simulink model "two_time_domains"  (R2025b)
settings: Solver=ode23tb  StartTime=0.0  StopTime=simlength  MaxStep=tc
undefined symbols (not defined in the file): D1, omega_base, P, time_gain_afe_module_1, time_gain_afe_module_2, time_gain_inv_module_2, trgo_th_generator, ts_afe, ts_inv
settings Model: Creator=dbagn  LastModifiedBy=dbagn
settings SolverCC: NumberNewtonIterations=3.0  ZeroCrossControl=DisableAll  AlgebraicLoopSolver=TrustRegion  SolverResetMethod=Robust  AutoInsertRateTranBlk=on
settings DataIOCC: SaveOutput=off  SignalLogging=off  DSMLogging=off  SaveTime=off  ReturnWorkspaceOutputs=off
settings OptimizationCC: ReuseModelBlockBuffer=off
settings DebuggingCC: UnconnectedInputMsg=warning  UnconnectedOutputMsg=warning  UnconnectedLineMsg=warning
settings ModelReferenceCC: UpdateModelReferenceTargets=Force  EnableRefExpFcnMdlSchedulingChecks=on  ParallelModelReferenceMATLABWorkerInit=Copy Base Workspace
settings SFSimCC: CustomCodeUndefinedFunction=ThrowError  DefaultCustomCodeDeterministicFunctions=All
settings RTWCC: GPUComputeCapability=3.5  DLArmComputeVersion=19.05

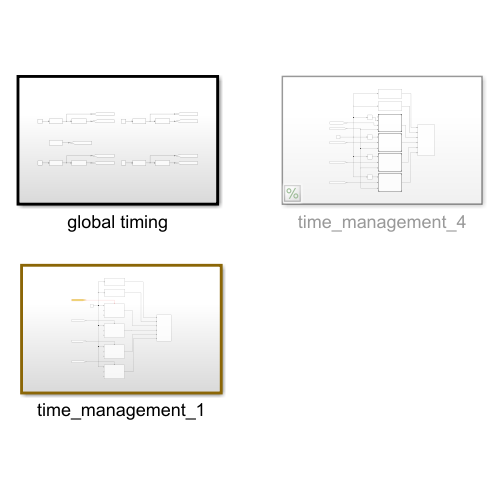
[thumbnail: Simulink's stored preview of the top-level diagram]
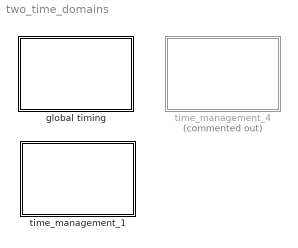
== system two_time_domains ==
  global timing : Subsystem
  time_management_1 : Subsystem
  time_management_4 : Subsystem  Commented=on

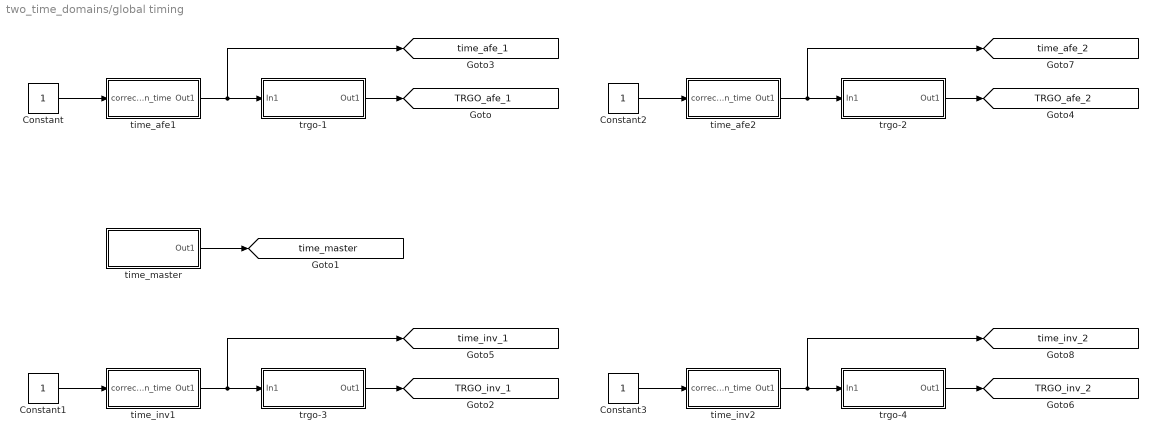
== system two_time_domains/global timing ==
  Constant{,1..3} (4 alike) : Constant
  time_afe1 : Subsystem  mask{k=time_gain_afe_module_1}
      mask prompts: k "Time Gain"
      mask Display:
      | disp('time-gen');
      | port_label('input', 1, 'crt');
      | port_label('output', 1, 'tout');
  time_afe2 : Subsystem  mask{k=time_gain_afe_module_2}
      mask prompts: k "Time Gain"
      mask Display:
      | disp('time-gen');
      | port_label('input', 1, 'crt');
      | port_label('output', 1, 'tout');
  time_inv1 : Subsystem  mask{k=time_gain_afe_module_1}
      mask prompts: k "Time Gain"
      mask Display:
      | disp('time-gen');
      | port_label('input', 1, 'crt');
      | port_label('output', 1, 'tout');
  time_inv2 : Subsystem  mask{k=time_gain_inv_module_2}
      mask prompts: k "Time Gain"
      mask Display:
      | disp('time-gen');
      | port_label('input', 1, 'crt');
      | port_label('output', 1, 'tout');
  time_master : Subsystem  mask{k=1}
      mask prompts: k "Time Gain"
      mask Display:
      | disp('master');
      | port_label('output', 1, 'time');
  trgo-1 : Subsystem  mask{samplig_time=ts_afe}
      mask prompts: samplig_time "Sampling Time"
      mask Display: disp('TRGO Generator');
  trgo-2 : Subsystem  mask{samplig_time=ts_afe}
      mask prompts: samplig_time "Sampling Time"
      mask Display: disp('TRGO Generator');
  trgo-3 : Subsystem  mask{samplig_time=ts_inv}
      mask prompts: samplig_time "Sampling Time"
      mask Display: disp('TRGO Generator');
  trgo-4 : Subsystem  mask{samplig_time=ts_inv}
      mask prompts: samplig_time "Sampling Time"
      mask Display: disp('TRGO Generator');
  tag scope: TRGO_afe_1=global, TRGO_afe_2=global, TRGO_inv_1=global, TRGO_inv_2=global, time_afe_1=global, time_afe_2=global, time_inv_1=global, time_inv_2=global, time_master=global
  wires:
  Constant/1 -> time_afe1/1(correction_time)
  time_afe1/1(Out1) -> [time_afe_1], trgo-1/1(In1)
  trgo-1/1(Out1) -> [TRGO_afe_1]
  trgo-2/1(Out1) -> [TRGO_afe_2]
  time_afe2/1(Out1) -> trgo-2/1(In1), [time_afe_2]
  Constant2/1 -> time_afe2/1(correction_time)
  time_master/1(Out1) -> [time_master]
  Constant3/1 -> time_inv2/1(correction_time)
  time_inv2/1(Out1) -> [time_inv_2], trgo-4/1(In1)
  trgo-4/1(Out1) -> [TRGO_inv_2]
  trgo-3/1(Out1) -> [TRGO_inv_1]
  time_inv1/1(Out1) -> trgo-3/1(In1), [time_inv_1]
  Constant1/1 -> time_inv1/1(correction_time)

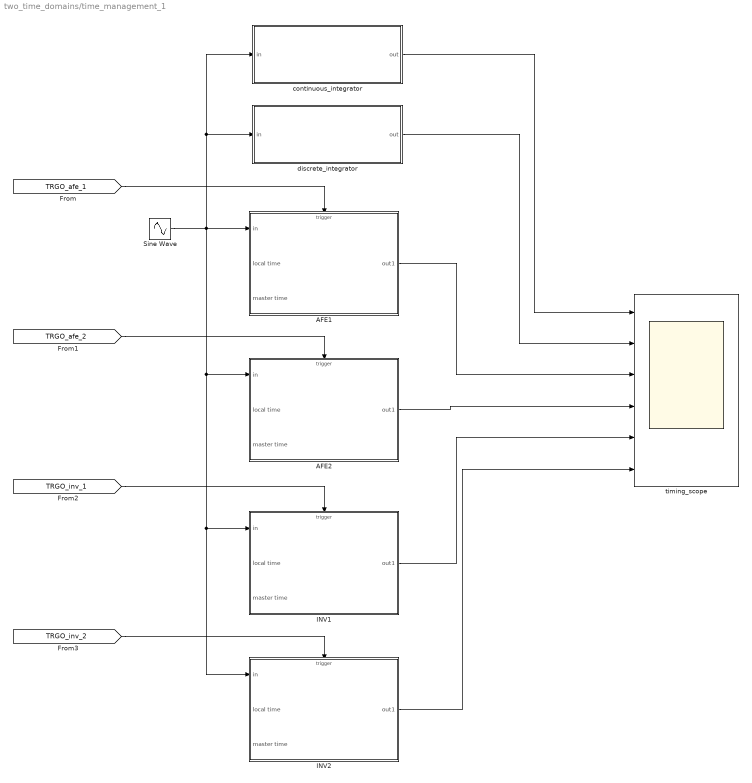
== system two_time_domains/time_management_1 ==
  AFE1 : Subsystem
  AFE2 : Subsystem
  INV1 : Subsystem
  INV2 : Subsystem
  Sine Wave : Sin  Frequency=omega_base  SampleTime=0
  continuous_integrator : Subsystem
  discrete_integrator : Subsystem
  timing_scope : Scope  NumInputPorts=6
      settings: SampleTime=tc  ActiveDisplayYMinimum=-0.51142077441090428  ActiveDisplayYMaximum=2.52734484585139
  wires:
  [TRGO_afe_1] -> AFE1/Trigger
  [TRGO_afe_2] -> AFE2/Trigger
  Sine Wave/1 -> discrete_integrator/1(in), continuous_integrator/1(in), AFE1/1(in), AFE2/1(in), INV2/1(in), INV1/1(in)
  [TRGO_inv_2] -> INV2/Trigger
  [TRGO_inv_1] -> INV1/Trigger
  AFE1/1(out1) -> timing_scope/3
  AFE2/1(out1) -> timing_scope/4
  INV1/1(out1) -> timing_scope/5
  INV2/1(out1) -> timing_scope/6
  discrete_integrator/1(out) -> timing_scope/2
  continuous_integrator/1(out) -> timing_scope/1

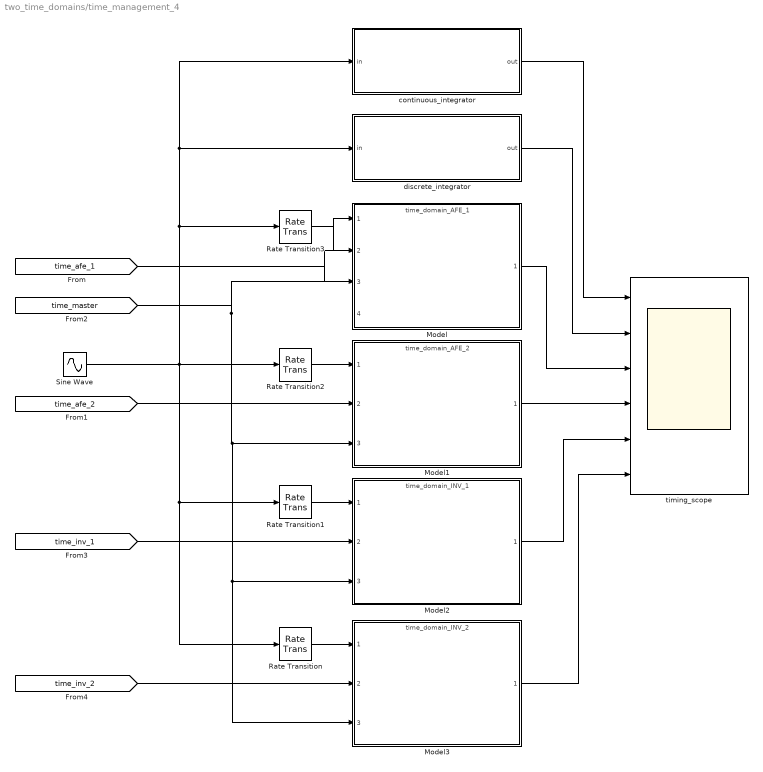
== system two_time_domains/time_management_4 ==
  Model : ModelReference  ModelNameDialog=time_domain_AFE_1  SimulationMode=Normal  ScheduleRates=on  CachedPortDiscreteRates=[0.00014000000000000001]  ModelEventPortInfo=P:D1[0.00014000000000000001][0][0]  ModelReferenceVersion=1.18  CommunicationStepSize=ts_afe_1
  Model1 : ModelReference  ModelNameDialog=time_domain_AFE_2  SimulationMode=Normal  ModelReferenceVersion=1.16  CommunicationStepSize=ts_afe_2
  Model2 : ModelReference  ModelNameDialog=time_domain_INV_1  SimulationMode=Normal  ModelReferenceVersion=1.19  CommunicationStepSize=ts_afe_1
  Model3 : ModelReference  ModelNameDialog=time_domain_INV_2  SimulationMode=Normal  ModelReferenceVersion=1.18  CommunicationStepSize=ts_afe_2
  Rate Transition : RateTransition  OutPortSampleTime=ts_inv_2
  Rate Transition1 : RateTransition  OutPortSampleTime=ts_inv_1
  Rate Transition2 : RateTransition  OutPortSampleTime=ts_afe_2
  Rate Transition3 : RateTransition  OutPortSampleTime=ts_afe_1
  Sine Wave : Sin  Frequency=omega_base  SampleTime=0
  continuous_integrator : Subsystem
  discrete_integrator : Subsystem
  timing_scope : Scope  NumInputPorts=6
      settings: SampleTime=tc  ActiveDisplayYMinimum=-0.24998930779814185  ActiveDisplayYMaximum=2.2499037701832774
  wires:
  Model/1 -> timing_scope/3
  Model1/1 -> timing_scope/4
  discrete_integrator/1(out) -> timing_scope/2
  [time_afe_1] -> Model/2
  [time_afe_2] -> Model1/2
  [time_master] -> Model3/3, Model2/3, Model1/3, Model/3
  Model2/1 -> timing_scope/5
  Model3/1 -> timing_scope/6
  Sine Wave/1 -> Rate Transition/1, Rate Transition1/1, discrete_integrator/1(in), continuous_integrator/1(in), Rate Transition3/1, Rate Transition2/1
  Rate Transition/1 -> Model3/1
  Rate Transition1/1 -> Model2/1
  Rate Transition2/1 -> Model1/1
  Rate Transition3/1 -> Model/1
  [time_inv_1] -> Model2/2
  [time_inv_2] -> Model3/2
  continuous_integrator/1(out) -> timing_scope/1

== system two_time_domains/global timing/time_afe1 ==
  correction_time : Inport
  Gain : Gain  Gain=k
  Product : Product
  time_1 : Clock
  Out1 : Outport
  wires:
  time_1/1 -> Gain/1
  Gain/1 -> Product/2
  Product/1 -> Out1/1
  correction_time/1 -> Product/1

== system two_time_domains/global timing/time_afe2 ==
  correction_time : Inport
  Gain : Gain  Gain=k
  Product : Product
  time_1 : Clock
  Out1 : Outport
  wires:
  correction_time/1 -> Product/1
  Product/1 -> Out1/1
  Gain/1 -> Product/2
  time_1/1 -> Gain/1

== system two_time_domains/global timing/time_inv1 ==
  correction_time : Inport
  Gain : Gain  Gain=k
  Product : Product
  time_1 : Clock
  Out1 : Outport
  wires:
  correction_time/1 -> Product/1
  Product/1 -> Out1/1
  Gain/1 -> Product/2
  time_1/1 -> Gain/1

== system two_time_domains/global timing/time_inv2 ==
  correction_time : Inport
  Gain : Gain  Gain=k
  Product : Product
  time_1 : Clock
  Out1 : Outport
  wires:
  time_1/1 -> Gain/1
  Gain/1 -> Product/2
  Product/1 -> Out1/1
  correction_time/1 -> Product/1

== system two_time_domains/global timing/time_master ==
  Gain : Gain  Gain=k
  time_1 : Clock
  Out1 : Outport
  wires:
  Gain/1 -> Out1/1
  time_1/1 -> Gain/1

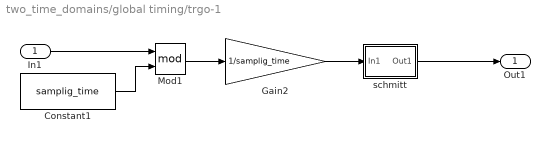
== system two_time_domains/global timing/trgo-1 ==
  In1 : Inport
  Constant1 : Constant  Value=samplig_time
  Gain2 : Gain  Gain=1/samplig_time
  Mod1 : Math  Operator=mod
  schmitt : Subsystem
  Out1 : Outport
  wires:
  Constant1/1 -> Mod1/2
  In1/1 -> Mod1/1
  Mod1/1 -> Gain2/1
  schmitt/1(Out1) -> Out1/1
  Gain2/1 -> schmitt/1(In1)

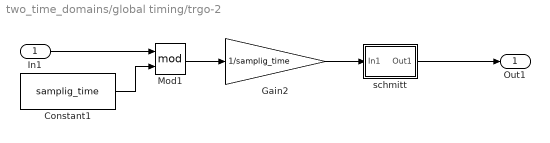
== system two_time_domains/global timing/trgo-2 ==
  In1 : Inport
  Constant1 : Constant  Value=samplig_time
  Gain2 : Gain  Gain=1/samplig_time
  Mod1 : Math  Operator=mod
  schmitt : Subsystem
  Out1 : Outport
  wires:
  Gain2/1 -> schmitt/1(In1)
  schmitt/1(Out1) -> Out1/1
  Mod1/1 -> Gain2/1
  In1/1 -> Mod1/1
  Constant1/1 -> Mod1/2

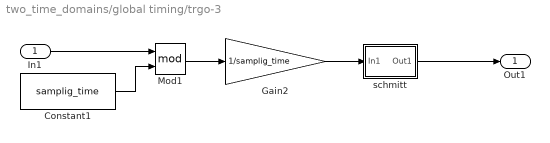
== system two_time_domains/global timing/trgo-3 ==
  In1 : Inport
  Constant1 : Constant  Value=samplig_time
  Gain2 : Gain  Gain=1/samplig_time
  Mod1 : Math  Operator=mod
  schmitt : Subsystem
  Out1 : Outport
  wires:
  Gain2/1 -> schmitt/1(In1)
  schmitt/1(Out1) -> Out1/1
  Mod1/1 -> Gain2/1
  In1/1 -> Mod1/1
  Constant1/1 -> Mod1/2

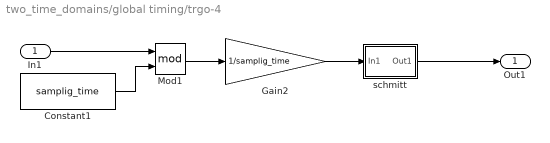
== system two_time_domains/global timing/trgo-4 ==
  In1 : Inport
  Constant1 : Constant  Value=samplig_time
  Gain2 : Gain  Gain=1/samplig_time
  Mod1 : Math  Operator=mod
  schmitt : Subsystem
  Out1 : Outport
  wires:
  Constant1/1 -> Mod1/2
  In1/1 -> Mod1/1
  Mod1/1 -> Gain2/1
  schmitt/1(Out1) -> Out1/1
  Gain2/1 -> schmitt/1(In1)

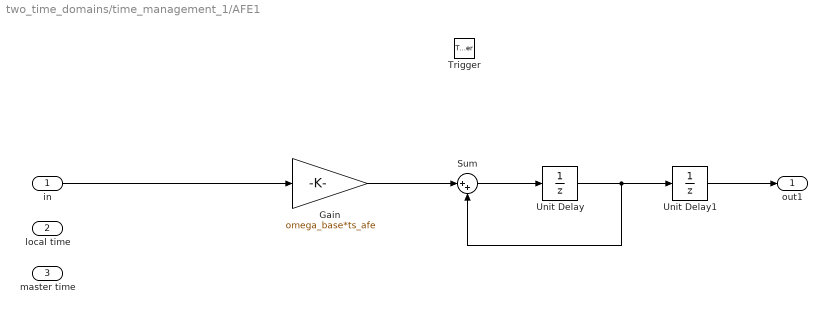
== system two_time_domains/time_management_1/AFE1 ==
  in : Inport
  local time : Inport  Port=2
  master time : Inport  Port=3
  Trigger : TriggerPort  VariantControl=(inherit)  PortDimensions=1
  Gain : Gain  Gain=omega_base*ts_afe
  Sum : Sum  Inputs=|++
  Unit Delay : UnitDelay  SampleTime=-1  HasFrameUpgradeWarning=on
  Unit Delay1 : UnitDelay  SampleTime=-1  HasFrameUpgradeWarning=on
  out1 : Outport
  wires:
  Gain/1 -> Sum/1
  Sum/1 -> Unit Delay/1
  Unit Delay/1 -> Sum/2, Unit Delay1/1
  in/1 -> Gain/1
  Unit Delay1/1 -> out1/1

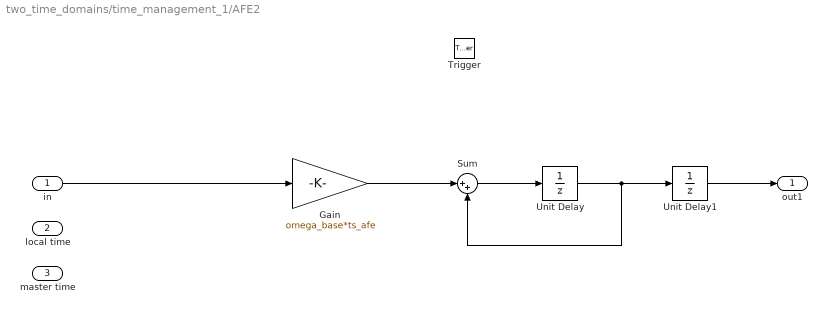
== system two_time_domains/time_management_1/AFE2 ==
  in : Inport
  local time : Inport  Port=2
  master time : Inport  Port=3
  Trigger : TriggerPort  VariantControl=(inherit)  PortDimensions=1
  Gain : Gain  Gain=omega_base*ts_afe
  Sum : Sum  Inputs=|++
  Unit Delay : UnitDelay  SampleTime=-1  HasFrameUpgradeWarning=on
  Unit Delay1 : UnitDelay  SampleTime=-1  HasFrameUpgradeWarning=on
  out1 : Outport
  wires:
  Unit Delay1/1 -> out1/1
  in/1 -> Gain/1
  Unit Delay/1 -> Unit Delay1/1, Sum/2
  Sum/1 -> Unit Delay/1
  Gain/1 -> Sum/1

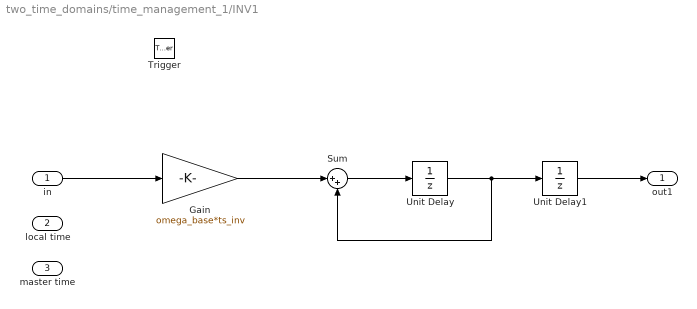
== system two_time_domains/time_management_1/INV1 ==
  in : Inport
  local time : Inport  Port=2
  master time : Inport  Port=3
  Trigger : TriggerPort  VariantControl=(inherit)  PortDimensions=1
  Gain : Gain  Gain=omega_base*ts_inv
  Sum : Sum  Inputs=|++
  Unit Delay : UnitDelay  SampleTime=-1  HasFrameUpgradeWarning=on
  Unit Delay1 : UnitDelay  SampleTime=-1  HasFrameUpgradeWarning=on
  out1 : Outport
  wires:
  Unit Delay1/1 -> out1/1
  in/1 -> Gain/1
  Unit Delay/1 -> Unit Delay1/1, Sum/2
  Sum/1 -> Unit Delay/1
  Gain/1 -> Sum/1

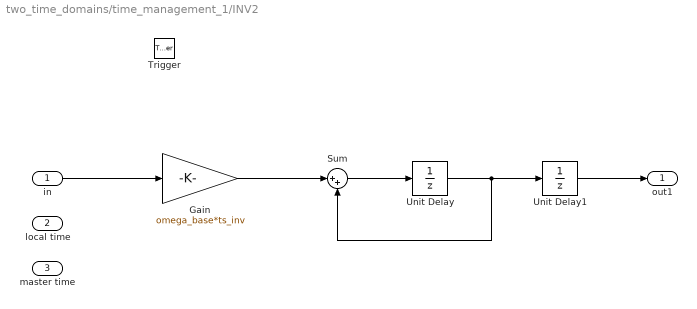
== system two_time_domains/time_management_1/INV2 ==
  in : Inport
  local time : Inport  Port=2
  master time : Inport  Port=3
  Trigger : TriggerPort  VariantControl=(inherit)  PortDimensions=1
  Gain : Gain  Gain=omega_base*ts_inv
  Sum : Sum  Inputs=|++
  Unit Delay : UnitDelay  SampleTime=-1  HasFrameUpgradeWarning=on
  Unit Delay1 : UnitDelay  SampleTime=-1  HasFrameUpgradeWarning=on
  out1 : Outport
  wires:
  Gain/1 -> Sum/1
  Sum/1 -> Unit Delay/1
  Unit Delay/1 -> Sum/2, Unit Delay1/1
  in/1 -> Gain/1
  Unit Delay1/1 -> out1/1

== system two_time_domains/time_management_1/continuous_integrator ==
  in : Inport
  Gain : Gain  Gain=omega_base
  Integrator : Integrator
  out : Outport
  wires:
  Integrator/1 -> out/1
  Gain/1 -> Integrator/1
  in/1 -> Gain/1

== system two_time_domains/time_management_1/discrete_integrator ==
  in : Inport
  Gain : Gain  Gain=omega_base*ts_afe
  Sum : Sum  Inputs=|++
  Unit Delay : UnitDelay  SampleTime=ts_afe  HasFrameUpgradeWarning=on
  Unit Delay1 : UnitDelay  SampleTime=ts_afe  HasFrameUpgradeWarning=on
  out : Outport
  wires:
  in/1 -> Gain/1
  Unit Delay1/1 -> out/1
  Gain/1 -> Sum/1
  Unit Delay/1 -> Unit Delay1/1, Sum/2
  Sum/1 -> Unit Delay/1

== system two_time_domains/time_management_4/continuous_integrator ==
  in : Inport
  Gain : Gain  Gain=omega_base
  Integrator : Integrator
  out : Outport
  wires:
  in/1 -> Gain/1
  Gain/1 -> Integrator/1
  Integrator/1 -> out/1

== system two_time_domains/time_management_4/discrete_integrator ==
  in : Inport
  Gain : Gain  Gain=omega_base*ts_afe
  Sum : Sum  Inputs=|++
  Unit Delay : UnitDelay  SampleTime=ts_afe  HasFrameUpgradeWarning=on
  Unit Delay1 : UnitDelay  SampleTime=ts_afe  HasFrameUpgradeWarning=on
  out : Outport
  wires:
  Sum/1 -> Unit Delay/1
  Unit Delay/1 -> Sum/2, Unit Delay1/1
  Gain/1 -> Sum/1
  Unit Delay1/1 -> out/1
  in/1 -> Gain/1

== system two_time_domains/global timing/trgo-1/schmitt ==
  In1 : Inport
  Constant2 : Constant
  Constant3 : Constant  Value=0
  Switch : Switch  Threshold=trgo_th_generator  SaturateOnIntegerOverflow=off  InputSameDT=off
  Out1 : Outport
  wires:
  Constant2/1 -> Switch/3
  Constant3/1 -> Switch/1
  In1/1 -> Switch/2
  Switch/1 -> Out1/1

== system two_time_domains/global timing/trgo-2/schmitt ==
  In1 : Inport
  Constant2 : Constant
  Constant3 : Constant  Value=0
  Switch : Switch  Threshold=trgo_th_generator  SaturateOnIntegerOverflow=off  InputSameDT=off
  Out1 : Outport
  wires:
  Switch/1 -> Out1/1
  In1/1 -> Switch/2
  Constant3/1 -> Switch/1
  Constant2/1 -> Switch/3

== system two_time_domains/global timing/trgo-3/schmitt ==
  In1 : Inport
  Constant2 : Constant
  Constant3 : Constant  Value=0
  Switch : Switch  Threshold=trgo_th_generator  SaturateOnIntegerOverflow=off  InputSameDT=off
  Out1 : Outport
  wires:
  Switch/1 -> Out1/1
  In1/1 -> Switch/2
  Constant3/1 -> Switch/1
  Constant2/1 -> Switch/3

== system two_time_domains/global timing/trgo-4/schmitt ==
  In1 : Inport
  Constant2 : Constant
  Constant3 : Constant  Value=0
  Switch : Switch  Threshold=trgo_th_generator  SaturateOnIntegerOverflow=off  InputSameDT=off
  Out1 : Outport
  wires:
  Constant2/1 -> Switch/3
  Constant3/1 -> Switch/1
  In1/1 -> Switch/2
  Switch/1 -> Out1/1
